simulink model "CI_Test"  (R2017a)
settings: Solver=ode3  StartTime=0.0  StopTime=10.0  RelTol=1e-3
settings Model: Creator=cac32742  LastModifiedBy=cac32742

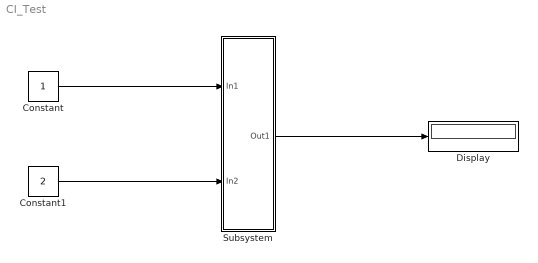
== system CI_Test ==
  Constant : Constant
  Constant1 : Constant  Value=2
  Display : Display
  Subsystem : Subsystem
  wires:
  Constant/1 -> Subsystem/1(In1)
  Constant1/1 -> Subsystem/2(In2)
  Subsystem/1(Out1) -> Display/1

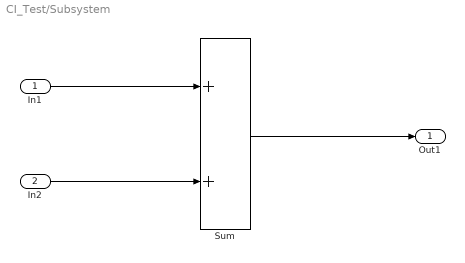
== system CI_Test/Subsystem ==
  In1 : Inport
  In2 : Inport  Port=2
  Sum : Sum
  Out1 : Outport
  wires:
  Sum/1 -> Out1/1
  In2/1 -> Sum/2
  In1/1 -> Sum/1
